simulink model "Arduino_Robot_model"  (R2015a)
settings: Solver=ode3  StartTime=0.0  StopTime=inf  RelTol=1e-3
libraries: arduinolib x8, simulink x1
settings Model: ExtModeTrigDuration=2  Creator=Chris  LastModifiedBy=Chris
settings OptimizationCC: OptimizeModelRefInitCode=on  LifeSpan=1
settings DebuggingCC: UnderspecifiedInitializationDetection=Classic  MergeDetectMultiDrivingBlocksExec=none  InheritedTsInSrcMsg=none
settings HardwareCC: ProdBitPerInt=16  ProdBitPerPointer=8  ProdIntDivRoundTo=Zero  ProdEndianess=LittleEndian  ProdWordSize=8  ProdHWDeviceType=Atmel->AVR
settings RTWCC: SystemTargetFile=realtime.tlc  GenerateMakefile=off  TemplateMakefile=realtime.tmf  Description=Run on Target Hardware  RTWVerbose=off
settings ERTTargetCC: CombineOutputUpdateFcns=off  ExtModeTransport=3  ExtModeMexFile=ext_serial_win32_comm_rtt  ExtModeMexArgs=0 1 9600  ERTSrcFileBannerTemplate=realtime_code_template.cgt  ERTHdrFileBannerTemplate=realtime_code_template.cgt  ERTDataSrcFileTemplate=realtime_code_template.cgt  ERTDataHdrFileTemplate=realtime_code_template.cgt  ERTCustomFileTemplate=realtime_file_process.tlc

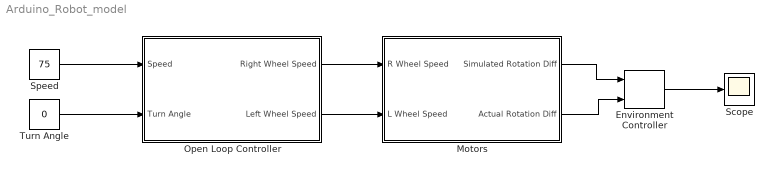
== system Arduino_Robot_model ==
  Environment Controller : simulink/Signal Routing/Environment Controller
  Motors : Subsystem
  Open Loop Controller : Subsystem
  Scope : Scope
  Speed : Constant  Value=75
  Turn Angle : Constant  Value=0
  wires:
  Speed/1 -> Open Loop Controller/1(Speed)
  Turn Angle/1 -> Open Loop Controller/2(Turn Angle)
  Open Loop Controller/1(Right Wheel Speed) -> Motors/1(R Wheel Speed)
  Open Loop Controller/2(Left Wheel Speed) -> Motors/2(L Wheel Speed)
  Motors/1(Simulated Rotation Diff) -> Environment Controller/1
  Motors/2(Actual Rotation Diff) -> Environment Controller/2
  Environment Controller/1 -> Scope/1

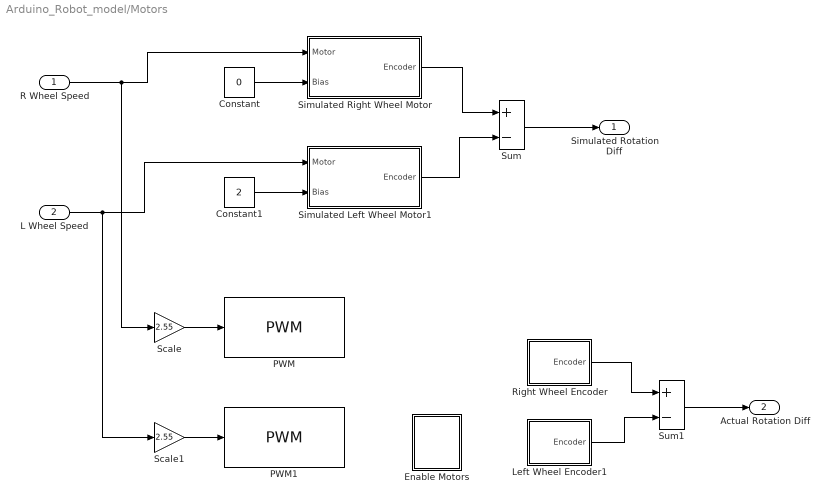
== system Arduino_Robot_model/Motors ==
  R Wheel Speed : Inport
  L Wheel Speed : Inport  Port=2
  Constant : Constant  Value=0  OutDataTypeStr=single
  Constant1 : Constant  Value=2  OutDataTypeStr=single
  Enable Motors : Subsystem
  Left Wheel Encoder1 : Subsystem
  PWM : arduinolib/PWM  pinNumber=10  blockPlatform=arduino
  PWM1 : arduinolib/PWM  pinNumber=11  blockPlatform=arduino
  Right Wheel Encoder : Subsystem
  Scale : Gain  Gain=2.55
  Scale1 : Gain  Gain=2.55
  Simulated Left Wheel Motor1 : Subsystem
  Simulated Right Wheel Motor : Subsystem
  Sum : Sum  Inputs=+-  OutDataTypeStr=Inherit: Same as first input
  Sum1 : Sum  Inputs=+-  OutDataTypeStr=Inherit: Same as first input
  Simulated Rotation Diff : Outport
  Actual Rotation Diff : Outport  Port=2
  wires:
  Constant/1 -> Simulated Right Wheel Motor/2(Bias)
  Constant1/1 -> Simulated Left Wheel Motor1/2(Bias)
  R Wheel Speed/1 -> Scale/1, Simulated Right Wheel Motor/1(Motor)
  L Wheel Speed/1 -> Simulated Left Wheel Motor1/1(Motor), Scale1/1
  Sum/1 -> Simulated Rotation Diff/1
  Simulated Right Wheel Motor/1(Encoder) -> Sum/1
  Simulated Left Wheel Motor1/1(Encoder) -> Sum/2
  Sum1/1 -> Actual Rotation Diff/1
  Right Wheel Encoder/1(Encoder) -> Sum1/1
  Left Wheel Encoder1/1(Encoder) -> Sum1/2
  Scale/1 -> PWM/1
  Scale1/1 -> PWM1/1

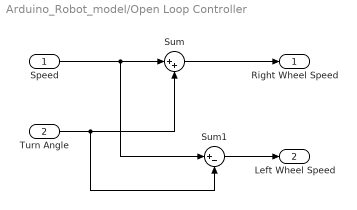
== system Arduino_Robot_model/Open Loop Controller ==
  Speed : Inport
  Turn Angle : Inport  Port=2
  Sum : Sum  Inputs=|++
  Sum1 : Sum  Inputs=|+-
  Right Wheel Speed : Outport
  Left Wheel Speed : Outport  Port=2
  wires:
  Speed/1 -> Sum1/1, Sum/1
  Sum/1 -> Right Wheel Speed/1
  Turn Angle/1 -> Sum/2, Sum1/2
  Sum1/1 -> Left Wheel Speed/1

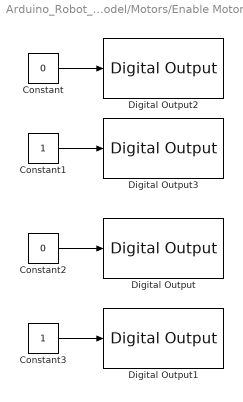
== system Arduino_Robot_model/Motors/Enable Motors ==
  Constant : Constant  Value=0  OutDataTypeStr=boolean
  Constant1 : Constant  OutDataTypeStr=boolean
  Constant2 : Constant  Value=0  OutDataTypeStr=boolean
  Constant3 : Constant  OutDataTypeStr=boolean
  Digital Output : arduinolib/Digital Output  pinNumber=2  blockPlatform=arduino
  Digital Output1 : arduinolib/Digital Output  pinNumber=3  blockPlatform=arduino
  Digital Output2 : arduinolib/Digital Output  pinNumber=4  blockPlatform=arduino
  Digital Output3 : arduinolib/Digital Output  pinNumber=5  blockPlatform=arduino
  wires:
  Constant1/1 -> Digital Output3/1
  Constant/1 -> Digital Output2/1
  Constant2/1 -> Digital Output/1
  Constant3/1 -> Digital Output1/1

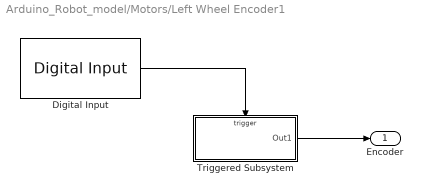
== system Arduino_Robot_model/Motors/Left Wheel Encoder1 ==
  Digital Input : arduinolib/Digital Input  pinNumber=9  sampleTime=1  blockPlatform=arduino
  Triggered Subsystem : Subsystem  TreatAsAtomicUnit=on
  Encoder : Outport
  wires:
  Digital Input/1 -> Triggered Subsystem/Trigger
  Triggered Subsystem/1(Out1) -> Encoder/1

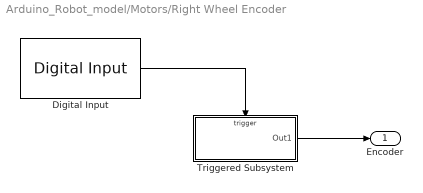
== system Arduino_Robot_model/Motors/Right Wheel Encoder ==
  Digital Input : arduinolib/Digital Input  pinNumber=8  sampleTime=1  blockPlatform=arduino
  Triggered Subsystem : Subsystem  TreatAsAtomicUnit=on
  Encoder : Outport
  wires:
  Digital Input/1 -> Triggered Subsystem/Trigger
  Triggered Subsystem/1(Out1) -> Encoder/1

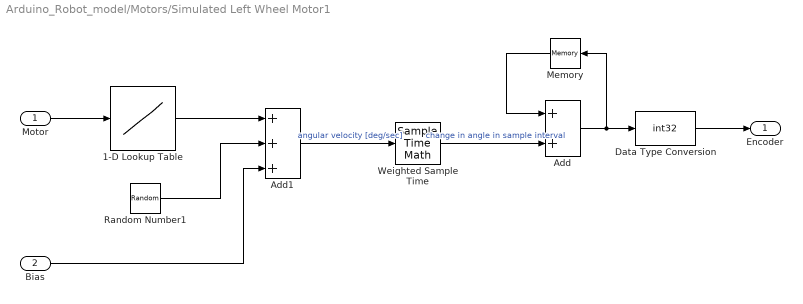
== system Arduino_Robot_model/Motors/Simulated Left Wheel Motor1 ==
  Motor : Inport
  Bias : Inport  Port=2
  1-D Lookup Table : Lookup_n-D  NumberOfTableDimensions=1  BreakpointsForDimension1=[-100 0 100]  Table=[-360 0 360]  ExtrapMethod=Clip  UseLastTableValue=on  RndMeth=Simplest  InputSameDT=on
  Add : Sum  OutDataTypeStr=Inherit: Same as first input
  Add1 : Sum  Inputs=+++  OutDataTypeStr=single
  Data Type Conversion : DataTypeConversion  OutDataTypeStr=int32
  Memory : Memory  InheritSampleTime=on  LinearizeAsDelay=on
  Random Number1 : RandomNumber  Variance=5  Seed=randi(1000)
  Weighted Sample Time : SampleTimeMath  TsampMathOp=*
  Encoder : Outport
  wires:
  Motor/1 -> 1-D Lookup Table/1
  1-D Lookup Table/1 -> Add1/1
  Random Number1/1 -> Add1/2
  Bias/1 -> Add1/3
  Add1/1 -> Weighted Sample Time/1  "angular velocity [deg/sec]"
  Weighted Sample Time/1 -> Add/2  "change in angle in sample interval"
  Add/1 -> Memory/1, Data Type Conversion/1
  Data Type Conversion/1 -> Encoder/1
  Memory/1 -> Add/1

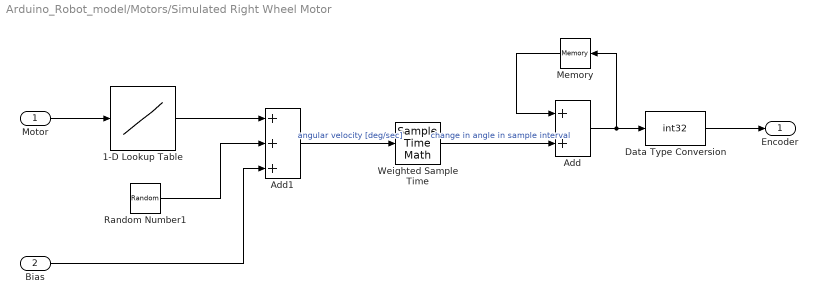
== system Arduino_Robot_model/Motors/Simulated Right Wheel Motor ==
  Motor : Inport
  Bias : Inport  Port=2
  1-D Lookup Table : Lookup_n-D  NumberOfTableDimensions=1  BreakpointsForDimension1=[-100 0 100]  Table=[-360 0 360]  ExtrapMethod=Clip  UseLastTableValue=on  RndMeth=Simplest  InputSameDT=on
  Add : Sum  OutDataTypeStr=Inherit: Same as first input
  Add1 : Sum  Inputs=+++  OutDataTypeStr=single
  Data Type Conversion : DataTypeConversion  OutDataTypeStr=int32
  Memory : Memory  InheritSampleTime=on  LinearizeAsDelay=on
  Random Number1 : RandomNumber  Variance=5  Seed=randi(1000)
  Weighted Sample Time : SampleTimeMath  TsampMathOp=*
  Encoder : Outport
  wires:
  Motor/1 -> 1-D Lookup Table/1
  1-D Lookup Table/1 -> Add1/1
  Random Number1/1 -> Add1/2
  Bias/1 -> Add1/3
  Add1/1 -> Weighted Sample Time/1  "angular velocity [deg/sec]"
  Weighted Sample Time/1 -> Add/2  "change in angle in sample interval"
  Add/1 -> Memory/1, Data Type Conversion/1
  Data Type Conversion/1 -> Encoder/1
  Memory/1 -> Add/1

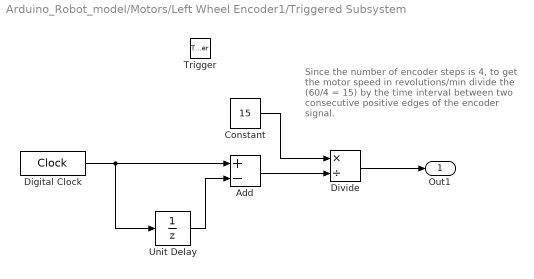
== system Arduino_Robot_model/Motors/Left Wheel Encoder1/Triggered Subsystem ==
  note: Since the number of encoder steps is 4,
      | to get the motor speed in revolutions/min
      | divide the (60/4 = 15) by the time interval
      | between two consecutive positive edges
      | of the encoder signal.
  Trigger : TriggerPort
  Add : Sum  Inputs=+-
  Constant : Constant  Value=15
  Digital Clock : DigitalClock  SampleTime=-1
  Divide : Product  Inputs=*/  OutDataTypeStr=int32
  Unit Delay : UnitDelay  SampleTime=-1
  Out1 : Outport
  wires:
  Digital Clock/1 -> Add/1, Unit Delay/1
  Unit Delay/1 -> Add/2
  Add/1 -> Divide/2
  Divide/1 -> Out1/1
  Constant/1 -> Divide/1

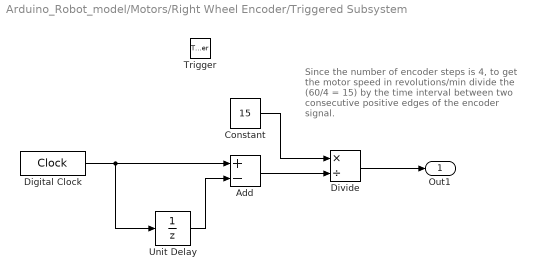
== system Arduino_Robot_model/Motors/Right Wheel Encoder/Triggered Subsystem ==
  note: Since the number of encoder steps is 4,
      | to get the motor speed in revolutions/min
      | divide the (60/4 = 15) by the time interval
      | between two consecutive positive edges
      | of the encoder signal.
  Trigger : TriggerPort
  Add : Sum  Inputs=+-
  Constant : Constant  Value=15
  Digital Clock : DigitalClock  SampleTime=-1
  Divide : Product  Inputs=*/  OutDataTypeStr=int32
  Unit Delay : UnitDelay  SampleTime=-1
  Out1 : Outport
  wires:
  Digital Clock/1 -> Add/1, Unit Delay/1
  Unit Delay/1 -> Add/2
  Add/1 -> Divide/2
  Divide/1 -> Out1/1
  Constant/1 -> Divide/1
